simulink model "MFTiresLongitudinalRearSSC"  (R2026b)
settings: Solver=VariableStepAuto
undefined symbols (not defined in the file): AxlTrq, BrkPrs, Fx, Fz, Kappa, Omega, PlntWhlDampCoeffRear, Vx
libraries: fl_lib x8, nesl_utility_internal x5, sdl_lib x2
settings Model: ModifiedByFormat=The MathWorks, Inc.  Creator=The MathWorks, Inc.  LastModifiedBy=The MathWorks, Inc.
settings OptimizationCC: ReuseModelBlockBuffer=off
settings DebuggingCC: SubsystemReferenceDiagnosticForUnitTest=warning
settings SimscapeCC: SimscapeUseEnergyAccounting=off

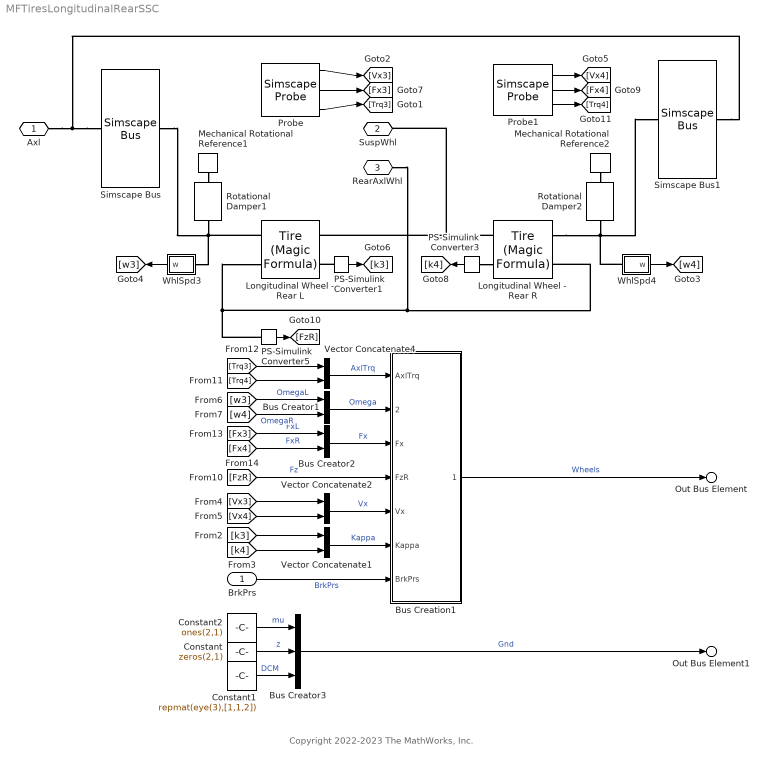
== system MFTiresLongitudinalRearSSC ==
  note: Copyright 2022-2023 The MathWorks, Inc.
  BrkPrs : Inport
  Bus Creator1 : BusCreator  Inputs=2
  Bus Creator2 : BusCreator  Inputs=2
  Bus Creator3 : BusCreator  Inputs=3
  Bus Creation1 : Subsystem
  Constant : Constant  Value=zeros(2,1)  SampleTime=-1
  Constant1 : Constant  Value=repmat(eye(3),[1,1,2])  SampleTime=-1
  Constant2 : Constant  Value=ones(2,1)  SampleTime=-1
  Longitudinal Wheel - Rear L : sdl_lib/Tires & Vehicles/Tire (Magic Formula)  parameterization=sdl.enum.magic_tire_model.constant  F_z1=3000 N  F_x1=3500 N  kappa1=10  B_m=PlntWhlLongStfFctrRear  C_m=PlntWhlLongShapeFctrRear  D_m=PlntWhlLongPeakFctrRear  E_m=PlntWhlLongCuvFctrRear  fz0=4000 N  p_Cx=1.685  p_Dx=[1.21, -.037]  p_Ex=[.344, .095, -.02, 0]  p_Kx=[21.51, -.163, .245]  p_Hx=[-.002, .002]  p_Vx=[0, 0]  rolling_radius_model=sdl.enum.RollingRadiusParameterization.Constant  r_e=PlntWhlLdRadiusRear m  r_0=0.3 m  breff=8.39  dreff=0.26  freff=0.074  q_re0=0.99  q_v1=0.008  longvl=17 m/s  cz=5e5 N/m  model_resistance=simscape.enum.onoff.on  resistance_model=sdl.enum.rollingResistanceParameterization.velocity  coeff=0.015  p_tire=PlntWhlPrsRear Pa  alpha=PlntWhlTirPrsExpRear  beta=PlntWhlNrmlForceExpRear  coeff_a=PlntWhlVelIndpntForceCffRear  coeff_b=PlntWhlLnrVelForceCompRear s/m  coeff_c=PlntWhlQuadVelForceCompRear s^2/m^2  p_tire0=240e3 Pa  fz0_resistance=4000 N  vH0=16 m/s  q_Sy=[.0082, 0, .0014, .001, 0, 0, 1.08, -.5]  v_thr=PlntWhlRollResVelThreshRear m/s  enable_scaling_coefficients=false  lfzO=1  lcx=1  lmux=1  lex=1  lkx=1  lhx=1  lvx=1  lmy=1  model_compliance=sdl.enum.compliance.off  stiffness=PlntWhlCompStiff N/m  damping=PlntWhlCompDamp N*s/m  model_inertia=sdl.enum.model_inertia.on  inertia=PlntWhlInertiaRear kg*m^2  initial_velocity=PlntWhlInitVelRear rad/s  vxlow=PlntWhlVelTolLowVelRear m/s  v_tr_thr=PlntWhlVelThreshRear m/s  kpumin=PlntWhlMinSlipRatioRear  kpumax=PlntWhlMaxSlipRatioRear
  Longitudinal Wheel - Rear R : sdl_lib/Tires & Vehicles/Tire (Magic Formula)  parameterization=sdl.enum.magic_tire_model.constant  F_z1=3000 N  F_x1=3500 N  kappa1=10  B_m=PlntWhlLongStfFctrRear  C_m=PlntWhlLongShapeFctrRear  D_m=PlntWhlLongPeakFctrRear  E_m=PlntWhlLongCuvFctrRear  fz0=4000 N  p_Cx=1.685  p_Dx=[1.21, -.037]  p_Ex=[.344, .095, -.02, 0]  p_Kx=[21.51, -.163, .245]  p_Hx=[-.002, .002]  p_Vx=[0, 0]  rolling_radius_model=sdl.enum.RollingRadiusParameterization.Constant  r_e=PlntWhlLdRadiusRear m  r_0=0.3 m  breff=8.39  dreff=0.26  freff=0.074  q_re0=0.99  q_v1=0.008  longvl=17 m/s  cz=5e5 N/m  model_resistance=simscape.enum.onoff.on  resistance_model=sdl.enum.rollingResistanceParameterization.velocity  coeff=0.015  p_tire=PlntWhlPrsRear Pa  alpha=PlntWhlTirPrsExpRear  beta=PlntWhlNrmlForceExpRear  coeff_a=PlntWhlVelIndpntForceCffRear  coeff_b=PlntWhlLnrVelForceCompRear s/m  coeff_c=PlntWhlQuadVelForceCompRear s^2/m^2  p_tire0=240e3 Pa  fz0_resistance=4000 N  vH0=16 m/s  q_Sy=[.0082, 0, .0014, .001, 0, 0, 1.08, -.5]  v_thr=PlntWhlRollResVelThreshRear m/s  enable_scaling_coefficients=false  lfzO=1  lcx=1  lmux=1  lex=1  lkx=1  lhx=1  lvx=1  lmy=1  model_compliance=sdl.enum.compliance.off  stiffness=PlntWhlCompStiff N/m  damping=PlntWhlCompDamp N*s/m  model_inertia=sdl.enum.model_inertia.on  inertia=PlntWhlInertiaRear kg*m^2  initial_velocity=PlntWhlInitVelRear rad/s  vxlow=PlntWhlVelTolLowVelRear m/s  v_tr_thr=PlntWhlVelThreshRear m/s  kpumin=PlntWhlMinSlipRatioRear  kpumax=PlntWhlMaxSlipRatioRear
  Mechanical Rotational Reference1 : fl_lib/Mechanical/Rotational Elements/Mechanical Rotational Reference
  Mechanical Rotational Reference2 : fl_lib/Mechanical/Rotational Elements/Mechanical Rotational Reference
  PS-Simulink Converter1 : nesl_utility_internal/PS-Simulink Converter  PhysicalDomain=network_engine_domain  SubClassName=ps_output  LeftPortType=input  RightPortType=output  PseudoPeriodic=off  Frequencies=[]  VectorFormat=inherit  Unit=inherit  AffineConversion=off
  PS-Simulink Converter3 : nesl_utility_internal/PS-Simulink Converter  PhysicalDomain=network_engine_domain  SubClassName=ps_output  LeftPortType=input  RightPortType=output  PseudoPeriodic=off  Frequencies=[]  VectorFormat=inherit  Unit=inherit  AffineConversion=off
  PS-Simulink Converter5 : nesl_utility_internal/PS-Simulink Converter  PhysicalDomain=network_engine_domain  SubClassName=ps_output  LeftPortType=input  RightPortType=output  PseudoPeriodic=off  Frequencies=[]  VectorFormat=inherit  Unit=inherit  AffineConversion=off
  Probe : SimscapeProbe  BoundBlock=109  Variables="{\"tire_road_interaction.T.v\":{\"Probing\":\"ON\"},\"tire_road_interaction.f_tread\":{\"Probing\":\"ON\"},\"wheel_axle.t\":{\"Probing\":\"ON\"}}"
  Probe1 : SimscapeProbe  BoundBlock=110  Variables="{\"tire_road_interaction.T.v\":{\"Probing\":\"ON\"},\"tire_road_interaction.f_tread\":{\"Probing\":\"ON\"},\"wheel_axle.t\":{\"Probing\":\"ON\"}}"
  Rotational Damper1 : fl_lib/Mechanical/Rotational Elements/Rotational Damper  D=PlntWhlDampCoeffRear N*m*s/rad  w_specify=off  w_priority=None  w=0 rad/s  w_nominal_specify=off  w_nominal_value=1  w_nominal_unit=rad/s  t_specify=off  t_priority=None  t=0 N*m  t_nominal_specify=off  t_nominal_value=1  t_nominal_unit=N*m
  Rotational Damper2 : fl_lib/Mechanical/Rotational Elements/Rotational Damper  D=PlntWhlDampCoeffRear N*m*s/rad  w_specify=off  w_priority=None  w=0 rad/s  w_nominal_specify=off  w_nominal_value=1  w_nominal_unit=rad/s  t_specify=off  t_priority=None  t=0 N*m  t_nominal_specify=off  t_nominal_value=1  t_nominal_unit=N*m
  Simscape Bus : SimscapeBus  HierarchyStrings=AxlRL
  Simscape Bus1 : SimscapeBus  HierarchyStrings=AxlRR
  Vector Concatenate1 : Concatenate
  Vector Concatenate2 : Concatenate
  Vector Concatenate4 : Concatenate
  WhlSpd3 : Subsystem
  WhlSpd4 : Subsystem
  Axl : PMIOPort  Side=Left
  SuspWhl : PMIOPort  Port=2  Side=Left
  RearAxlWhl : PMIOPort  Port=3  Side=Left
  Out Bus Element : Outport  PortName=RearWheels  Element=Wheels
  Out Bus Element1 : Outport  PortName=RearWheels  Element=Gnd
  wires:
  PS-Simulink Converter5/1 -> [FzR]
  PS-Simulink Converter1/1 -> [k3]
  WhlSpd3/1(w) -> [w3]
  WhlSpd4/1(w) -> [w4]
  PS-Simulink Converter3/1 -> [k4]
  Bus Creation1/1(Wheels) -> Out Bus Element/1  "Wheels"
  Constant2/1 -> Bus Creator3/1  "mu"
  Constant/1 -> Bus Creator3/2  "z"
  Constant1/1 -> Bus Creator3/3  "DCM"
  Bus Creator3/1 -> Out Bus Element1/1  "Gnd"
  [Fx3] -> Bus Creator2/1  "FxL"
  Bus Creator2/1 -> Bus Creation1/3(Fx)  "Fx"
  [Trq4] -> Vector Concatenate4/2
  Vector Concatenate4/1 -> Bus Creation1/1(AxlTrq)  "AxlTrq"
  Vector Concatenate2/1 -> Bus Creation1/5(Vx)  "Vx"
  [Vx4] -> Vector Concatenate2/2
  [FzR] -> Bus Creation1/4(FzR)  "Fz"
  [Fx4] -> Bus Creator2/2  "FxR"
  [w3] -> Bus Creator1/1  "OmegaL"
  [k4] -> Vector Concatenate1/2
  Vector Concatenate1/1 -> Bus Creation1/6(Kappa)  "Kappa"
  Bus Creator1/1 -> Bus Creation1/2(Omega)  "Omega"
  [w4] -> Bus Creator1/2  "OmegaR"
  [Vx3] -> Vector Concatenate2/1
  [k3] -> Vector Concatenate1/1
  [Trq3] -> Vector Concatenate4/1
  BrkPrs/1 -> Bus Creation1/7(BrkPrs)  "BrkPrs"
  Probe/1 -> [Vx3]
  Probe1/2 -> [Fx4]
  Probe1/3 -> [Trq4]
  Probe/2 -> [Fx3]
  Probe/3 -> [Trq3]
  Probe1/1 -> [Vx4]
  connections:
  Longitudinal Wheel - Rear R/LConn1 -- Longitudinal Wheel - Rear L/LConn1 -- PS-Simulink Converter5/LConn1 -- RearAxlWhl/RConn1
  Longitudinal Wheel - Rear R/LConn2 -- Simscape Bus1/LConn1 -- Rotational Damper2/LConn1 -- WhlSpd4/LConn1
  Simscape Bus/RConn1 -- Simscape Bus1/RConn1 -- Axl/RConn1
  Simscape Bus/LConn1 -- Rotational Damper1/LConn1 -- Longitudinal Wheel - Rear L/LConn2 -- WhlSpd3/LConn1
  Longitudinal Wheel - Rear R/RConn2 -- SuspWhl/RConn1 -- Longitudinal Wheel - Rear L/RConn2
  PS-Simulink Converter1/LConn1 -- Longitudinal Wheel - Rear L/RConn1
  Mechanical Rotational Reference1/LConn1 -- Rotational Damper1/RConn1
  Mechanical Rotational Reference2/LConn1 -- Rotational Damper2/RConn1
  PS-Simulink Converter3/LConn1 -- Longitudinal Wheel - Rear R/RConn1

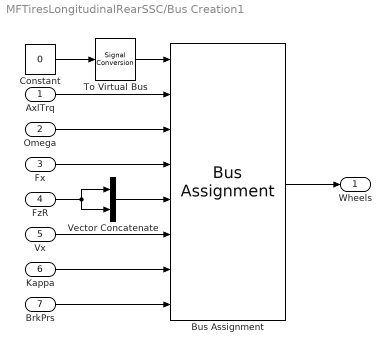
== system MFTiresLongitudinalRearSSC/Bus Creation1 ==
  AxlTrq : Inport
  Omega : Inport  Port=2
  Fx : Inport  Port=3
  FzR : Inport  Port=4
  Vx : Inport  Port=5
  Kappa : Inport  Port=6
  BrkPrs : Inport  Port=7
  Bus Assignment : BusAssignment  AssignedSignals=AxlTrq,Omega,Fx,Fz,Vx,Kappa,BrkPrs
  Constant : Constant  Value=0  OutDataTypeStr=Bus: RWheelsBUS  SampleTime=Inf
  To Virtual Bus : SignalConversion  ConversionOutput=Virtual bus  OverrideOpt=off
  Vector Concatenate : Concatenate
  Wheels : Outport
  wires:
  To Virtual Bus/1 -> Bus Assignment/1
  Bus Assignment/1 -> Wheels/1
  FzR/1 -> Vector Concatenate/1, Vector Concatenate/2
  Vector Concatenate/1 -> Bus Assignment/5
  Constant/1 -> To Virtual Bus/1
  Omega/1 -> Bus Assignment/3
  BrkPrs/1 -> Bus Assignment/8
  Kappa/1 -> Bus Assignment/7
  AxlTrq/1 -> Bus Assignment/2
  Vx/1 -> Bus Assignment/6
  Fx/1 -> Bus Assignment/4

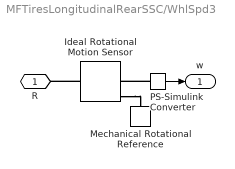
== system MFTiresLongitudinalRearSSC/WhlSpd3 ==
  Ideal Rotational Motion Sensor : fl_lib/Mechanical/Mechanical Sensors/Ideal Rotational Motion Sensor  reference=foundation.enum.MeasurementReference.difference  acceleration_port=false  velocity_port=true  position_port=true  wrap_angle=simscape.enum.onoff.off  offset=0 rad
  Mechanical Rotational Reference : fl_lib/Mechanical/Rotational Elements/Mechanical Rotational Reference
  PS-Simulink Converter : nesl_utility_internal/PS-Simulink Converter  PhysicalDomain=network_engine_domain  SubClassName=ps_output  LeftPortType=input  RightPortType=output  PseudoPeriodic=off  Frequencies=[]  VectorFormat=inherit  Unit=inherit  AffineConversion=off
  R : PMIOPort  Side=Left
  w : Outport
  wires:
  PS-Simulink Converter/1 -> w/1
  connections:
  PS-Simulink Converter/LConn1 -- Ideal Rotational Motion Sensor/RConn2
  Ideal Rotational Motion Sensor/LConn1 -- R/RConn1
  Ideal Rotational Motion Sensor/RConn1 -- Mechanical Rotational Reference/LConn1

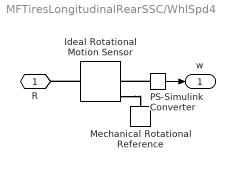
== system MFTiresLongitudinalRearSSC/WhlSpd4 ==
  Ideal Rotational Motion Sensor : fl_lib/Mechanical/Mechanical Sensors/Ideal Rotational Motion Sensor  reference=foundation.enum.MeasurementReference.difference  acceleration_port=false  velocity_port=true  position_port=true  wrap_angle=simscape.enum.onoff.off  offset=0 rad
  Mechanical Rotational Reference : fl_lib/Mechanical/Rotational Elements/Mechanical Rotational Reference
  PS-Simulink Converter : nesl_utility_internal/PS-Simulink Converter  PhysicalDomain=network_engine_domain  SubClassName=ps_output  LeftPortType=input  RightPortType=output  PseudoPeriodic=off  Frequencies=[]  VectorFormat=inherit  Unit=inherit  AffineConversion=off
  R : PMIOPort  Side=Left
  w : Outport
  wires:
  PS-Simulink Converter/1 -> w/1
  connections:
  Ideal Rotational Motion Sensor/RConn1 -- Mechanical Rotational Reference/LConn1
  Ideal Rotational Motion Sensor/LConn1 -- R/RConn1
  PS-Simulink Converter/LConn1 -- Ideal Rotational Motion Sensor/RConn2
